simulink model "drive_AC1"  (R2015a)
settings: Solver=FixedStepDiscrete  StartTime=0.0  StopTime=4.5  RelTol=1e-3
PreLoadFcn:
  | Ts=20e-6;
libraries: powerlib_meascontrol x6, powerlib x2, electricdrivelib x1
Description:
  | Copyright 2008-2015 The MathWorks, Inc.
settings Model: CovSFcnEnable=off  ExtModeAutoUpdateStatusClock=off  Creator=MathWorks  LastModifiedBy=range
settings DataIOCC: SignalLoggingName=sigsOut
settings OptimizationCC: ExpressionDepthLimit=2147483647  InitFltsAndDblsToZero=on
settings DebuggingCC: UnderspecifiedInitializationDetection=Classic  MergeDetectMultiDrivingBlocksExec=none  CheckExecutionContextPreStartOutputMsg=on  CheckExecutionContextRuntimeOutputMsg=on  SignalResolutionControl=TryResolveAllWithWarning  MultiTaskDSMMsg=warning  MultiTaskCondExecSysMsg=none  FcnCallInpInsideContextMsg=UseLocalSettings  StateNameClashWarn=warning
settings HardwareCC: TargetUnknown=on
settings GRTTargetCC: CombineOutputUpdateFcns=off  GRTInterface=on
settings SimscapeCC: SimscapeLogType=all  SimscapeLogDataHistory=10000

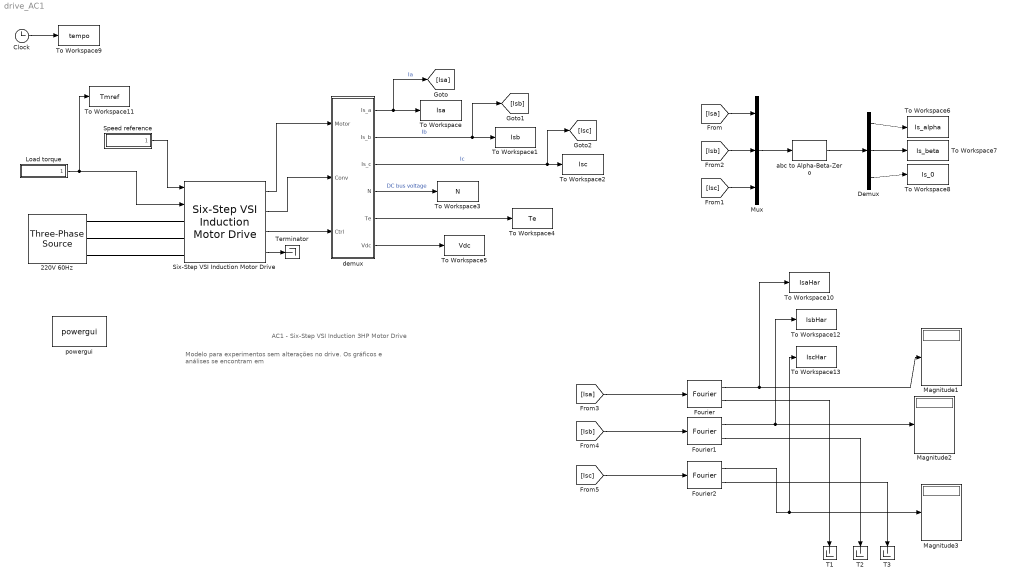
== system drive_AC1 ==
  note: Modelo para experimentos sem alterações no drive.
      | Os gráficos e análises se encontram em
  note: AC1 - Six-Step VSI Induction 3HP Motor Drive
  220V 60Hz : powerlib/Electrical Sources/Three-Phase Source  Voltage=220  PhaseAngle=0  Frequency=60  InternalConnection=Yg  SpecifyImpedance=off  Resistance=0.1  Inductance=0.1e-3  ShortCircuitLevel=0  BaseVoltage=0  XRratio=0  BusType=swing  Pref=0  Qref=0  Qmin=-inf  Qmax=inf
  Clock : Clock
  Demux : Demux  Outputs=3
  Fourier : powerlib_meascontrol/Measurements/Fourier  Freq=60  n=[0:20]  InInit=[0, 0]  Ts=Ts
  Fourier1 : powerlib_meascontrol/Measurements/Fourier  Freq=60  n=[0:20]  InInit=[0, 0]  Ts=Ts
  Fourier2 : powerlib_meascontrol/Measurements/Fourier  Freq=60  n=[0:20]  InInit=[0, 0]  Ts=Ts
  Load torque : Subsystem
  Magnitude1 : Display
      settings: Format=bank
  Magnitude2 : Display
      settings: Format=bank
  Magnitude3 : Display
      settings: Format=bank
  Mux : Mux  Inputs=3
  Six-Step VSI Induction Motor Drive : electricdrivelib/AC drives/Six-Step VSI Induction Motor Drive  showMaskWarnings=on  AverageValue=off  MechanicalLoad=Torque Tm  driveType=AC1  outputBusMode=Multiple output buses
  Speed reference : Subsystem
  T1 : Terminator
  T2 : Terminator
  T3 : Terminator
  Terminator : Terminator
  To Workspace : ToWorkspace  VariableName=Isa  SampleTime=-1
  To Workspace1 : ToWorkspace  VariableName=Isb  SampleTime=-1
  To Workspace10 : ToWorkspace  VariableName=IsaHar  SampleTime=-1
  To Workspace11 : ToWorkspace  VariableName=Tmref  SampleTime=-1
  To Workspace12 : ToWorkspace  VariableName=IsbHar  SampleTime=-1
  To Workspace13 : ToWorkspace  VariableName=IscHar  SampleTime=-1
  To Workspace2 : ToWorkspace  VariableName=Isc  SampleTime=-1
  To Workspace3 : ToWorkspace  VariableName=N  SampleTime=-1
  To Workspace4 : ToWorkspace  VariableName=Te  SampleTime=-1
  To Workspace5 : ToWorkspace  VariableName=Vdc  SampleTime=-1
  To Workspace6 : ToWorkspace  VariableName=Is_alpha  SampleTime=-1
  To Workspace7 : ToWorkspace  VariableName=Is_beta  SampleTime=-1
  To Workspace8 : ToWorkspace  VariableName=Is_0  SampleTime=-1
  To Workspace9 : ToWorkspace  VariableName=tempo  SampleTime=-1
  abc to Alpha-Beta-Zero : powerlib_meascontrol/Transformations/abc to Alpha-Beta-Zero
  demux : Subsystem
  powergui : powerlib/powergui  Priority=2  SimulationMode=Discrete  SolverType=Tustin/Backward Euler (TBE)  SampleTime=Ts  frequency=60  SPID=off  DisableSnubberDevices=off  DisableRonSwitches=off  DisableVfSwitches=off  SwTol=0  DisplayEquations=off  Interpol=off  methode=off  Ts=0  FunctionMessages=off  echomessages=off  HookPort=off  EnableUseOfTLC=off  x0status=blocks  frequencyindice=60  Pbase=100e6  ErrMax=1e-4  Iterations=50  UnitsV=kV  UnitsW=MW  buscounter=0  RestoreLinks=warning  ResistiveCurrentMeasurement=off  Frange=[0:2:500]  Ylog=off  Xlog=on  ShowGrid=off  save=off  variable=ZData  structure=0  ZoomFFT=on  StartTime=0.0  cycles=1  DisplayStyle=1  fundamental=60  FreqAxis=off  MaxFrequency=1000  frequencyindicesteady=1  RmsSteady=1  display=off
  wires:
  Speed reference/1(" ") -> Six-Step VSI Induction Motor Drive/1
  Load torque/1(" ") -> To Workspace11/1, Six-Step VSI Induction Motor Drive/2
  Six-Step VSI Induction Motor Drive/1 -> demux/1(Motor)
  Six-Step VSI Induction Motor Drive/2 -> demux/2(Conv)
  Six-Step VSI Induction Motor Drive/3 -> demux/3(Ctrl)
  Six-Step VSI Induction Motor Drive/4 -> Terminator/1
  demux/1(Is_a) -> To Workspace/1, [Isa]  "Ia"
  demux/2(Is_b) -> To Workspace1/1, [Isb]  "Ib"
  demux/3(Is_c) -> To Workspace2/1, [Isc]  "Ic"
  demux/4(N) -> To Workspace3/1  "DC bus voltage"
  demux/5(Te) -> To Workspace4/1
  demux/6(Vdc) -> To Workspace5/1
  Mux/1 -> abc to Alpha-Beta-Zero/1
  [Isa] -> Mux/1
  [Isb] -> Mux/2
  [Isc] -> Mux/3
  abc to Alpha-Beta-Zero/1 -> Demux/1
  Demux/1 -> To Workspace6/1
  Demux/2 -> To Workspace7/1
  Demux/3 -> To Workspace8/1
  Clock/1 -> To Workspace9/1
  [Isa] -> Fourier/1
  Fourier/1 -> To Workspace10/1, Magnitude1/1
  Fourier/2 -> T1/1
  Fourier1/2 -> T2/1
  Fourier2/2 -> T3/1
  [Isb] -> Fourier1/1
  [Isc] -> Fourier2/1
  Fourier1/1 -> To Workspace12/1, Magnitude2/1
  Fourier2/1 -> To Workspace13/1, Magnitude3/1
  connections:
  220V 60Hz/RConn1 -- Six-Step VSI Induction Motor Drive/LConn1
  220V 60Hz/RConn2 -- Six-Step VSI Induction Motor Drive/LConn2
  220V 60Hz/RConn3 -- Six-Step VSI Induction Motor Drive/LConn3

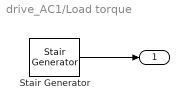
== system drive_AC1/Load torque ==
  Stair Generator : powerlib_meascontrol/Pulse & Signal Generators/Stair Generator  t=[0. 1.]  e=[0. 7.7]  Ts=Ts
  " " : Outport
  wires:
  Stair Generator/1 -> " "/1

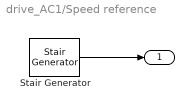
== system drive_AC1/Speed reference ==
  Stair Generator : powerlib_meascontrol/Pulse & Signal Generators/Stair Generator  t=[0]  e=[1800]  Ts=Ts
  " " : Outport
  wires:
  Stair Generator/1 -> " "/1

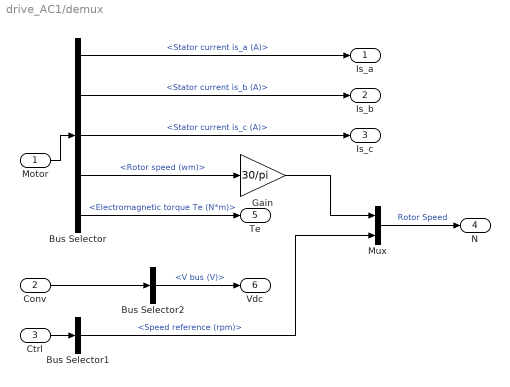
== system drive_AC1/demux ==
  Motor : Inport
  Conv : Inport  Port=2
  Ctrl : Inport  Port=3
  Bus Selector : BusSelector  OutputSignals=Stator measurements.Stator current is_a (A),Stator measurements.Stator current is_b (A),Stator measurements.Stator current is_c (A),Mechanical.Rotor speed (wm),Mechanical.Electromagnetic torque Te (N*m)
  Bus Selector1 : BusSelector  OutputSignals=Speed reference (rpm)
  Bus Selector2 : BusSelector  OutputSignals=V bus (V)
  Gain : Gain  Gain=30/pi  SaturateOnIntegerOverflow=on  OutDataTypeStr=Inherit: Same as input  ParamDataTypeStr=Inherit: Same as input
  Mux : Mux  Inputs=2
  Is_a : Outport
  Is_b : Outport  Port=2
  Is_c : Outport  Port=3
  N : Outport  Port=4
  Te : Outport  Port=5
  Vdc : Outport  Port=6
  wires:
  Bus Selector/4 -> Gain/1  "<Rotor speed (wm)>"
  Gain/1 -> Mux/1
  Bus Selector1/1 -> Mux/2  "<Speed reference (rpm)>"
  Bus Selector/1 -> Is_a/1  "<Stator current is_a (A)>"
  Motor/1 -> Bus Selector/1
  Conv/1 -> Bus Selector2/1
  Ctrl/1 -> Bus Selector1/1
  Bus Selector/3 -> Is_c/1  "<Stator current is_c (A)>"
  Bus Selector/2 -> Is_b/1  "<Stator current is_b (A)>"
  Mux/1 -> N/1  "Rotor Speed"
  Bus Selector/5 -> Te/1  "<Electromagnetic torque Te (N*m)>"
  Bus Selector2/1 -> Vdc/1  "<V bus (V)>"
